simulink model "Sigma_Delta_NLDAC_DWA_RES_SL"  (Simulink 7.5)
settings: Solver=ode45  StartTime=0.0  StopTime=10.0  RelTol=1e-3
values from neighbouring files (symbols this model uses):
  a1 = 0.5019    [Loop_NLDAC.mat]    (also in Loop_NLDAC_BiDWA.mat; Sigma_Delta_Linear_DAC.m; Sigma_Delta_Linear_DAC_loop.m; Sigma_Delta_NLDAC.m)
  a2 = 0.3042    [Loop_NLDAC.mat]    (also in Loop_NLDAC_BiDWA.mat; Sigma_Delta_Linear_DAC.m; Sigma_Delta_Linear_DAC_loop.m; Sigma_Delta_NLDAC.m)
  alfa = 0.999    [Loop_NLDAC.mat]    (also in Loop_NLDAC_BiDWA.mat; Sigma_Delta_Linear_DAC.m; Sigma_Delta_Linear_DAC_loop.m; Sigma_Delta_NLDAC.m)
  Amax = 1.8    [Loop_NLDAC.mat]    (also in Loop_NLDAC_BiDWA.mat; Sigma_Delta_Linear_DAC.m; Sigma_Delta_Linear_DAC_loop.m; Sigma_Delta_NLDAC.m)
  Ampl = 0.19    [Loop_NLDAC.mat]    (also in Loop_NLDAC_BiDWA.mat; Sigma_Delta_Linear_DAC.m = 0.3; Sigma_Delta_Linear_DAC_loop.m; Sigma_Delta_NLDAC.m)
  b1 = 0.5019    [Loop_NLDAC.mat]    (also in Loop_NLDAC_BiDWA.mat; Sigma_Delta_Linear_DAC.m; Sigma_Delta_Linear_DAC_loop.m; Sigma_Delta_NLDAC.m)
  b2 = 0.3042    [Loop_NLDAC.mat]    (also in Loop_NLDAC_BiDWA.mat; Sigma_Delta_Linear_DAC.m; Sigma_Delta_Linear_DAC_loop.m; Sigma_Delta_NLDAC.m)
  b3 = 1    [Loop_NLDAC.mat]    (also in Loop_NLDAC_BiDWA.mat; Sigma_Delta_Linear_DAC.m = 0; Sigma_Delta_Linear_DAC_loop.m; Sigma_Delta_NLDAC.m)
  c1 = 0.2817    [Loop_NLDAC.mat]    (also in Loop_NLDAC_BiDWA.mat; Sigma_Delta_Linear_DAC.m; Sigma_Delta_Linear_DAC_loop.m; Sigma_Delta_NLDAC.m)
  c2 = 5.7104    [Loop_NLDAC.mat]    (also in Loop_NLDAC_BiDWA.mat; Sigma_Delta_Linear_DAC.m; Sigma_Delta_Linear_DAC_loop.m; Sigma_Delta_NLDAC.m)
  Cf = 2.5e-12    [Loop_NLDAC.mat]    (also in Loop_NLDAC_BiDWA.mat; Sigma_Delta_Linear_DAC.m; Sigma_Delta_Linear_DAC_loop.m; Sigma_Delta_NLDAC.m = 2.5)
  const = 0    [Loop_NLDAC.mat]    (also in Loop_NLDAC_BiDWA.mat; Sigma_Delta_Linear_DAC.m; Sigma_Delta_Linear_DAC_loop.m; Sigma_Delta_NLDAC.m)
  DAC_shift = 0.225    [Loop_NLDAC.mat]    (also in Loop_NLDAC_BiDWA.mat; Sigma_Delta_Linear_DAC.m; Sigma_Delta_Linear_DAC_loop.m; Sigma_Delta_NLDAC.m)
  finrad = 63.813600776    [Loop_NLDAC.mat]    (also in Loop_NLDAC_BiDWA.mat; Sigma_Delta_Linear_DAC.m = Fin*2*pi; Sigma_Delta_Linear_DAC_loop.m = Fin*2*pi; Sigma_Delta_NLDAC.m = Fin*2*pi)
  GBW = 4000000    [Loop_NLDAC.mat]    (also in Loop_NLDAC_BiDWA.mat; Sigma_Delta_Linear_DAC.m; Sigma_Delta_Linear_DAC_loop.m; Sigma_Delta_NLDAC.m)
  k = 1.38e-23    [Loop_NLDAC.mat]    (also in Loop_NLDAC_BiDWA.mat; Sigma_Delta_Linear_DAC.m; Sigma_Delta_Linear_DAC_loop.m; Sigma_Delta_NLDAC.m)
  noise1 = 3e-08    [Loop_NLDAC.mat]    (also in Loop_NLDAC_BiDWA.mat; Sigma_Delta_Linear_DAC.m; Sigma_Delta_Linear_DAC_loop.m; Sigma_Delta_NLDAC.m = 0)
  r1 = 0.5019    [Loop_NLDAC.mat]    (also in Loop_NLDAC_BiDWA.mat; Sigma_Delta_Linear_DAC.m; Sigma_Delta_Linear_DAC_loop.m; Sigma_Delta_NLDAC.m)
  r2 = 0.3042    [Loop_NLDAC.mat]    (also in Loop_NLDAC_BiDWA.mat; Sigma_Delta_Linear_DAC.m; Sigma_Delta_Linear_DAC_loop.m; Sigma_Delta_NLDAC.m)
  random = 0.1125    [Loop_NLDAC.mat]    (also in Loop_NLDAC_BiDWA.mat; Sigma_Delta_Linear_DAC.m; Sigma_Delta_Linear_DAC_loop.m; Sigma_Delta_NLDAC.m)
  sr = inf    [Loop_NLDAC.mat]    (also in Loop_NLDAC_BiDWA.mat; Sigma_Delta_Linear_DAC.m; Sigma_Delta_Linear_DAC_loop.m; Sigma_Delta_NLDAC.m)
  Temp = 300    [Loop_NLDAC.mat]    (also in Loop_NLDAC_BiDWA.mat; Sigma_Delta_Linear_DAC.m; Sigma_Delta_Linear_DAC_loop.m; Sigma_Delta_NLDAC.m)
  Ts = 1.953125e-05    [Loop_NLDAC.mat]    (also in Loop_NLDAC_BiDWA.mat; Sigma_Delta_Linear_DAC.m; Sigma_Delta_Linear_DAC_loop.m; Sigma_Delta_NLDAC.m)
  Ts_pn = Ts * 128    (= 0.0025)    [Sigma_Delta_NLDAC_DWA_RES.m]
  UEG0 = 0.225297400264    [Loop_NLDAC.mat]    (also in Loop_NLDAC_BiDWA.mat = 0.224094362454; Sigma_Delta_Linear_DAC_loop.m = DAC_step * ( 1 + frac_error(i,j,1) ); Sigma_Delta_NLDAC.m = DAC_step * ( 1 + frac_error(1) ); Sigma_Delta_NLDAC_BiDWA.m = DAC_step * ( 1 + frac_error(1) ))
  UEG1 = 0.225809869923    [Loop_NLDAC.mat]    (also in Loop_NLDAC_BiDWA.mat = 0.2240538032; Sigma_Delta_Linear_DAC_loop.m = DAC_step * ( 1 + frac_error(i,j,2) ); Sigma_Delta_NLDAC.m = DAC_step * ( 1 + frac_error(2) ); Sigma_Delta_NLDAC_BiDWA.m = DAC_step * ( 1 + frac_error(2) ))
  UEG2 = 0.224626431014    [Loop_NLDAC.mat]    (also in Loop_NLDAC_BiDWA.mat = 0.225728482718; Sigma_Delta_Linear_DAC_loop.m = DAC_step * ( 1 + frac_error(i,j,3) ); Sigma_Delta_NLDAC.m = DAC_step * ( 1 + frac_error(3) ); Sigma_Delta_NLDAC_BiDWA.m = DAC_step * ( 1 + frac_error(3) ))
  UEG3 = 0.225382310978    [Loop_NLDAC.mat]    (also in Loop_NLDAC_BiDWA.mat = 0.225896977376; Sigma_Delta_Linear_DAC_loop.m = DAC_step * ( 1 + frac_error(i,j,4) ); Sigma_Delta_NLDAC.m = DAC_step * ( 1 + frac_error(4) ); Sigma_Delta_NLDAC_BiDWA.m = DAC_step * ( 1 + frac_error(4) ))
  UEG4 = 0.225571027107    [Loop_NLDAC.mat]    (also in Loop_NLDAC_BiDWA.mat = 0.224420295179; Sigma_Delta_Linear_DAC_loop.m = DAC_step * ( 1 + frac_error(i,j,5) ); Sigma_Delta_NLDAC.m = DAC_step * ( 1 + frac_error(5) ); Sigma_Delta_NLDAC_BiDWA.m = DAC_step * ( 1 + frac_error(5) ))
  UEG5 = 0.225259624957    [Loop_NLDAC.mat]    (also in Loop_NLDAC_BiDWA.mat = 0.224828213498; Sigma_Delta_Linear_DAC_loop.m = DAC_step * ( 1 + frac_error(i,j,6) ); Sigma_Delta_NLDAC.m = DAC_step * ( 1 + frac_error(6) ); Sigma_Delta_NLDAC_BiDWA.m = DAC_step * ( 1 + frac_error(6) ))
  UEG6 = 0.224443920639    [Loop_NLDAC.mat]    (also in Loop_NLDAC_BiDWA.mat = 0.223228145386; Sigma_Delta_Linear_DAC_loop.m = DAC_step * ( 1 + frac_error(i,j,7) ); Sigma_Delta_NLDAC.m = DAC_step * ( 1 + frac_error(7) ); Sigma_Delta_NLDAC_BiDWA.m = DAC_step * ( 1 + frac_error(7) ))
  Vin_bias = 0.9    [Loop_NLDAC.mat]    (also in Loop_NLDAC_BiDWA.mat; Sigma_Delta_Linear_DAC.m; Sigma_Delta_Linear_DAC_loop.m; Sigma_Delta_NLDAC.m)
undefined symbols (not defined in the file or in its folder): clock, slew
libraries: simulink x8, commseqgen2 x2, simulink_extras x1
settings Model: Creator=test  LastModifiedBy=Mahmoud Sawaby

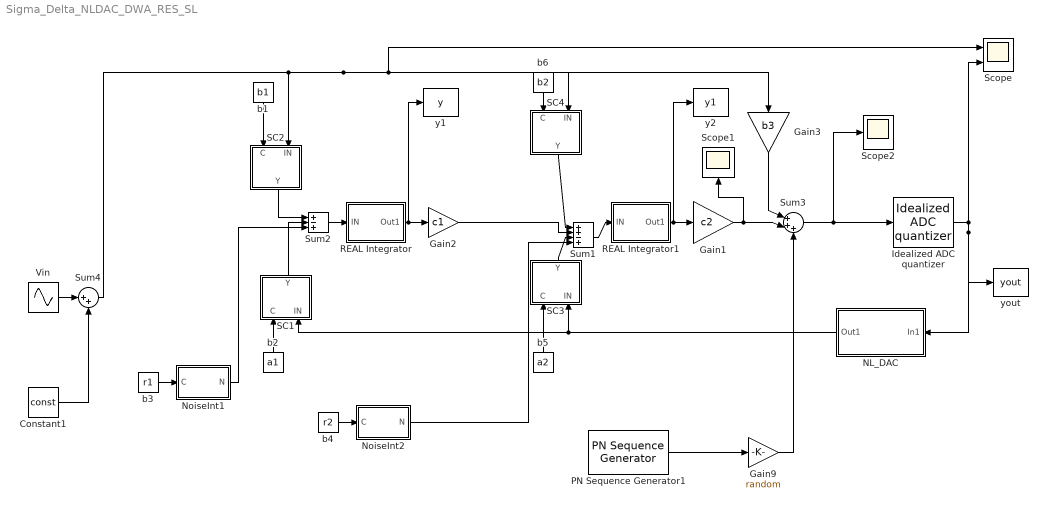
== system Sigma_Delta_NLDAC_DWA_RES_SL ==
  Constant1 : Constant  Value=const  OutDataType=fixdt(1, 16)  OutScaling=2^0  SampleTime=Ts
  Gain1 : Gain  Gain=c2  ParameterDataType=fixdt(1, 16)  ParameterScaling=2^0  OutDataType=fixdt(1, 16)  OutScaling=2^0
  Gain2 : Gain  Gain=c1  ParameterDataType=fixdt(1, 16)  ParameterScaling=2^0  OutDataType=fixdt(1, 16)  OutScaling=2^0
  Gain3 : Gain  Gain=b3  ParameterDataType=fixdt(1, 16)  ParameterScaling=2^0  OutDataType=fixdt(1, 16)  OutScaling=2^0
  Gain9 : Gain  Gain=random  ParameterDataType=fixdt(1, 16)  ParameterScaling=2^0  OutDataType=fixdt(1, 16)  OutScaling=2^0
  Idealized ADC quantizer : simulink_extras/Additional Discrete/Idealized ADC quantizer  SystemSampleTime=-1  NumberOfConverterBits=3  Vmin=MIN_volt  Vmax=MAX_volt  OutputDataType=double  OutputNegativeValues=off
  NL_DAC : Subsystem
  NoiseInt1 : Subsystem  mask(OpAmp Noise){seed=sum(clock)^1/111, Ts=Ts, noise=noise1}
      mask prompts: seed "Random Number Seed:"; Ts "Sample Time:"; noise "Op-amp Noise Std. Dev.:"
      mask Display: disp('OpNoise')
  NoiseInt2 : Subsystem  mask(OpAmp Noise){seed=sum(clock)^1/111, Ts=Ts, noise=noise1}
      mask prompts: seed "Random Number Seed:"; Ts "Sample Time:"; noise "Op-amp Noise Std. Dev.:"
      mask Display: disp('OpNoise')
  PN Sequence Generator1 : commseqgen2/PN Sequence Generator  poly=[1 0 0 0 0 0 0 0 0 0 0 1 0 1 1 0 1]  ini_sta=[0 0 0 0 0 0 0 0 0 0 0 0 0 0 0 1]  outBitMaskSource=Dialog parameter  shift=0  Ts=Ts  frameBased=off  sampPerFrame=18  reset=off  bitPackedOutputs=off  outDataType=double  numPackedBits=8  bitPackDataSigned=off  bitPackedOutDType=double
  REAL Integrator : Subsystem  mask(Integrator){Ts=Ts, alfa=alfa, Amax=Amax, sr=sr, GBW=GBW}
      mask prompts: Ts "Sample Time:"; alfa "Finite Gain:"; Amax "Saturation:"; sr "Slew Rate:"; GBW "Gain-Bandwidth"
      mask help:
      | Real discrete integrator with delay.
      | Models op-amp saturation and slew rate.
      mask Help:
      | Parameters:
      | Ts:       Sample time
      | G:         Finite op-amp gain (ideal op-amp G=1)
      | Amax:  Saturation value
      | sr:       slew rate in V/s
      mask Display: dpoly([0 1], [1 -1], 'z-')
  REAL Integrator1 : Subsystem  mask(Integrator){Ts=Ts, alfa=alfa, Amax=Amax, sr=sr, GBW=GBW}
      mask prompts: Ts "Sample Time:"; alfa "Finite Gain:"; Amax "Saturation:"; sr "Slew Rate:"; GBW "Gain-Bandwidth"
      mask help:
      | Real discrete integrator with delay.
      | Models op-amp saturation and slew rate.
      mask Help:
      | Parameters:
      | Ts:       Sample time
      | G:         Finite op-amp gain (ideal op-amp G=1)
      | Amax:  Saturation value
      | sr:       slew rate in V/s
      mask Display: dpoly([0 1], [1 -1], 'z-')
  SC1 : Subsystem  mask(kT/C Noise){Ts=Ts, Ci=Cf, Temp=Temp, k=k, seed=sum(clock)}
      mask prompts: Ts "Sample Time:"; Ci "Integrating Capacitance:"; Temp "Absolute Temperature:"; k "Boltzman Constant:"; seed "Random Number Seed:"
      mask help:
      | Models the kT/Cs noise of a switched capacitance Cs.
      | IN input: the input signal line
      | C input:   accepts the coefficient WITH SIGN (Cs/Ci)
      mask Help:
      | Block parameters:
      | Ts:        Sample time
      | Ci:        Integrating Capacitance
      | Temp:   Absolute Temperature in Kelvin
      | k:         Boltzmann Constant
      | seed:    Initial seed for random number generator
      | Outputs the noisy signal.
      mask Display: disp('kT/C')
  SC2 : Subsystem  mask(kT/C Noise){Ts=Ts, Ci=Cf, Temp=Temp, k=k, seed=sum(clock)}
      mask prompts: Ts "Sample Time:"; Ci "Integrating Capacitance:"; Temp "Absolute Temperature:"; k "Boltzman Constant:"; seed "Random Number Seed:"
      mask help:
      | Models the kT/Cs noise of a switched capacitance Cs.
      | IN input: the input signal line
      | C input:   accepts the coefficient WITH SIGN (Cs/Ci)
      mask Help:
      | Block parameters:
      | Ts:        Sample time
      | Ci:        Integrating Capacitance
      | Temp:   Absolute Temperature in Kelvin
      | k:         Boltzmann Constant
      | seed:    Initial seed for random number generator
      | Outputs the noisy signal.
      mask Display: disp('kT/C')
  SC3 : Subsystem  mask(kT/C Noise){Ts=Ts, Ci=Cf, Temp=Temp, k=k, seed=sum(clock)}
      mask prompts: Ts "Sample Time:"; Ci "Integrating Capacitance:"; Temp "Absolute Temperature:"; k "Boltzman Constant:"; seed "Random Number Seed:"
      mask help:
      | Models the kT/Cs noise of a switched capacitance Cs.
      | IN input: the input signal line
      | C input:   accepts the coefficient WITH SIGN (Cs/Ci)
      mask Help:
      | Block parameters:
      | Ts:        Sample time
      | Ci:        Integrating Capacitance
      | Temp:   Absolute Temperature in Kelvin
      | k:         Boltzmann Constant
      | seed:    Initial seed for random number generator
      | Outputs the noisy signal.
      mask Display: disp('kT/C')
  SC4 : Subsystem  mask(kT/C Noise){Ts=Ts, Ci=Cf, Temp=Temp, k=k, seed=sum(clock)}
      mask prompts: Ts "Sample Time:"; Ci "Integrating Capacitance:"; Temp "Absolute Temperature:"; k "Boltzman Constant:"; seed "Random Number Seed:"
      mask help:
      | Models the kT/Cs noise of a switched capacitance Cs.
      | IN input: the input signal line
      | C input:   accepts the coefficient WITH SIGN (Cs/Ci)
      mask Help:
      | Block parameters:
      | Ts:        Sample time
      | Ci:        Integrating Capacitance
      | Temp:   Absolute Temperature in Kelvin
      | k:         Boltzmann Constant
      | seed:    Initial seed for random number generator
      | Outputs the noisy signal.
      mask Display: disp('kT/C')
  Scope : Scope  NumInputPorts=2
      settings: YMin=0.1~-1  YMax=1.7~8  MaxDataPoints=65536
  Scope1 : Scope
  Scope2 : Scope
      settings: YMin=-0.5  YMax=2.4  SaveName=ScopeData2  MaxDataPoints=65536
  Sum1 : Sum  Inputs=++-+  SaturateOnIntegerOverflow=on  InputSameDT=on  OutDataTypeStr=Inherit: Same as first input
  Sum2 : Sum  Inputs=+-+  SaturateOnIntegerOverflow=on  InputSameDT=on  OutDataTypeStr=Inherit: Same as first input
  Sum3 : Sum  Inputs=|+++  OutDataType=fixdt(1, 16)  OutScaling=2^0
  Sum4 : Sum  Inputs=|++  OutDataType=fixdt(1, 16)  OutScaling=2^0
  Vin : Sin  Amplitude=Ampl  Bias=Vin_bias  Frequency=finrad  Phase=0  Samples=10  SampleTime=Ts  Offset=0
  b1 : Constant  Value=b1  SampleTime=Ts
  b2 : Constant  Value=a1  SampleTime=Ts
  b3 : Constant  Value=r1
  b4 : Constant  Value=r2
  b5 : Constant  Value=a2  SampleTime=Ts
  b6 : Constant  Value=b2  SampleTime=Ts
  y1 : ToWorkspace  VariableName=y  SampleTime=-1  SaveFormat=Array
  y2 : ToWorkspace  VariableName=y1  SampleTime=-1  SaveFormat=Array
  yout : ToWorkspace  VariableName=yout  SampleTime=Ts  SaveFormat=Array
  wires:
  Idealized ADC quantizer/1 -> yout/1, NL_DAC/1(In1), Scope/2
  Gain1/1 -> Scope1/1, Sum3/2
  REAL Integrator/1(Out1) -> y1/1, Gain2/1
  REAL Integrator1/1(Out1) -> Gain1/1, y2/1
  Sum2/1 -> REAL Integrator/1(IN)
  Sum3/1 -> Idealized ADC quantizer/1, Scope2/1
  Gain3/1 -> Sum3/1
  Sum4/1 -> Scope/1, Gain3/1, SC4/2(IN), SC2/2(IN)
  Constant1/1 -> Sum4/2
  Gain9/1 -> Sum3/3
  Vin/1 -> Sum4/1
  SC1/1(Y) -> Sum2/2
  b2/1 -> SC1/1(C)
  b1/1 -> SC2/1(C)
  SC2/1(Y) -> Sum2/1
  SC4/1(Y) -> Sum1/1
  Gain2/1 -> Sum1/2
  SC3/1(Y) -> Sum1/3
  Sum1/1 -> REAL Integrator1/1(IN)
  PN Sequence Generator1/1 -> Gain9/1
  b3/1 -> NoiseInt1/1(C)
  NoiseInt1/1(N) -> Sum2/3
  b4/1 -> NoiseInt2/1(C)
  b5/1 -> SC3/1(C)
  b6/1 -> SC4/1(C)
  NL_DAC/1(Out1) -> SC1/2(IN), SC3/2(IN)
  NoiseInt2/1(N) -> Sum1/4

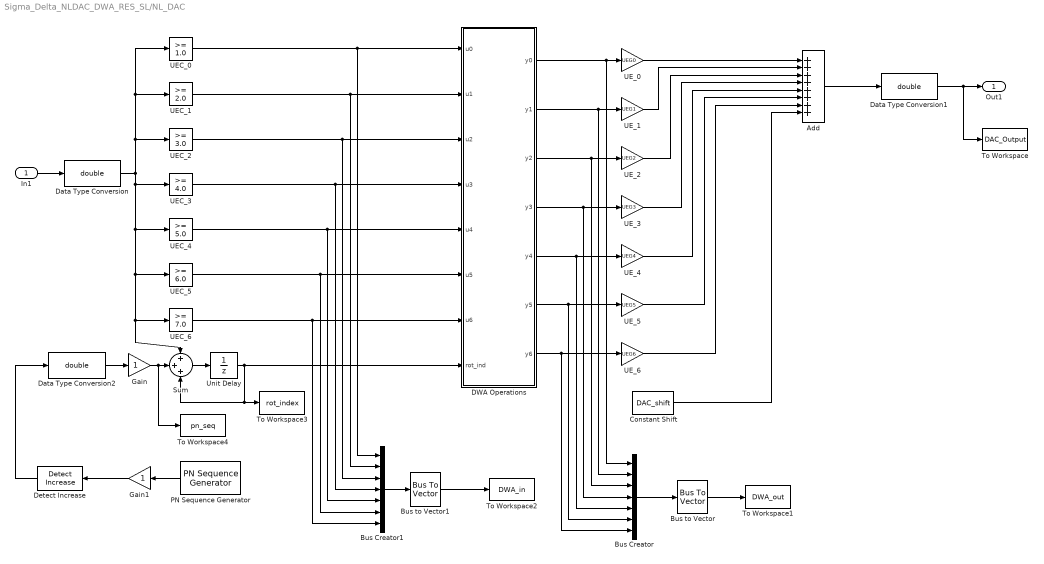
== system Sigma_Delta_NLDAC_DWA_RES_SL/NL_DAC ==
  In1 : Inport  OutDataType=fixdt(1, 16)  OutScaling=2^0
  Add : Sum  Inputs=++++++++  OutDataType=fixdt(1, 16)  OutScaling=2^-10
  Bus Creator : BusCreator  Inputs=7
  Bus Creator1 : BusCreator  Inputs=7
  Bus to Vector : BusToVector
  Bus to Vector1 : BusToVector
  Constant Shift : Constant  Value=DAC_shift  OutDataType=fixdt(1, 16)  OutScaling=2^0  SampleTime=Ts
  DWA Operations : Stateflow chart  TreatAsAtomicUnit=on  SystemSampleTime=Ts
  Data Type Conversion : DataTypeConversion  OutDataTypeMode=double  OutDataType=fixdt(1, 16)  OutScaling=2^0  OutDataTypeStr=double  SampleTime=Ts
  Data Type Conversion1 : DataTypeConversion  OutDataTypeMode=double  OutDataType=fixdt(1, 16)  OutScaling=2^0  OutDataTypeStr=double
  Data Type Conversion2 : DataTypeConversion  OutDataTypeMode=double  OutDataType=fixdt(1, 16)  OutScaling=2^0  OutDataTypeStr=double  SampleTime=Ts
  Detect Increase : simulink/Logic and Bit Operations/Detect Increase  SystemSampleTime=-1  vinit=0.0
  Gain : Gain  ParameterDataType=fixdt(1, 16)  ParameterScaling=2^0  OutDataType=fixdt(1, 16)  OutScaling=2^0
  Gain1 : Gain  ParameterDataType=fixdt(1, 16)  ParameterScaling=2^0  OutDataType=fixdt(1, 16)  OutScaling=2^0  SampleTime=Ts
  PN Sequence Generator : commseqgen2/PN Sequence Generator  poly=[6 5 0]  ini_sta=[0 0 0 0 0 1]  outBitMaskSource=Dialog parameter  shift=0  Ts=Ts_pn  frameBased=off  sampPerFrame=1  reset=off  bitPackedOutputs=off  outDataType=double  numPackedBits=8  bitPackDataSigned=off  bitPackedOutDType=double
  Sum : Sum  Inputs=+++  OutDataType=fixdt(1, 16)  OutScaling=2^0
  To Workspace : ToWorkspace  VariableName=DAC_Output  SampleTime=-1  SaveFormat=Array
  To Workspace1 : ToWorkspace  VariableName=DWA_out  SampleTime=-1  SaveFormat=Array
  To Workspace2 : ToWorkspace  VariableName=DWA_in  SampleTime=-1  SaveFormat=Array
  To Workspace3 : ToWorkspace  VariableName=rot_index  SampleTime=-1  SaveFormat=Array
  To Workspace4 : ToWorkspace  VariableName=pn_seq  SampleTime=-1  SaveFormat=Array
  UEC_0 : simulink/Logic and Bit Operations/Compare To Constant  SystemSampleTime=-1  relop=>=  const=1.0  LogicOutDataTypeMode=uint8
  UEC_1 : simulink/Logic and Bit Operations/Compare To Constant  SystemSampleTime=-1  relop=>=  const=2.0  LogicOutDataTypeMode=uint8
  UEC_2 : simulink/Logic and Bit Operations/Compare To Constant  SystemSampleTime=-1  relop=>=  const=3.0  LogicOutDataTypeMode=uint8
  UEC_3 : simulink/Logic and Bit Operations/Compare To Constant  SystemSampleTime=-1  relop=>=  const=4.0  LogicOutDataTypeMode=uint8
  UEC_4 : simulink/Logic and Bit Operations/Compare To Constant  SystemSampleTime=-1  relop=>=  const=5.0  LogicOutDataTypeMode=uint8
  UEC_5 : simulink/Logic and Bit Operations/Compare To Constant  SystemSampleTime=-1  relop=>=  const=6.0  LogicOutDataTypeMode=uint8
  UEC_6 : simulink/Logic and Bit Operations/Compare To Constant  SystemSampleTime=-1  relop=>=  const=7.0  LogicOutDataTypeMode=uint8
  UE_0 : Gain  Gain=UEG0  ParameterDataType=fixdt(1, 16)  ParameterScaling=2^0  OutDataType=fixdt(1, 16)  OutScaling=2^0
  UE_1 : Gain  Gain=UEG1  ParameterDataType=fixdt(1, 16)  ParameterScaling=2^0  OutDataType=fixdt(1, 16)  OutScaling=2^0
  UE_2 : Gain  Gain=UEG2  ParameterDataType=fixdt(1, 16)  ParameterScaling=2^0  OutDataType=fixdt(1, 16)  OutScaling=2^0
  UE_3 : Gain  Gain=UEG3  ParameterDataType=fixdt(1, 16)  ParameterScaling=2^0  OutDataType=fixdt(1, 16)  OutScaling=2^0
  UE_4 : Gain  Gain=UEG4  ParameterDataType=fixdt(1, 16)  ParameterScaling=2^0  OutDataType=fixdt(1, 16)  OutScaling=2^0
  UE_5 : Gain  Gain=UEG5  ParameterDataType=fixdt(1, 16)  ParameterScaling=2^0  OutDataType=fixdt(1, 16)  OutScaling=2^0
  UE_6 : Gain  Gain=UEG6  ParameterDataType=fixdt(1, 16)  ParameterScaling=2^0  OutDataType=fixdt(1, 16)  OutScaling=2^0
  Unit Delay : UnitDelay  SampleTime=-1
  Out1 : Outport  OutDataType=fixdt(1, 16)  OutScaling=2^0
  wires:
  UE_0/1 -> Add/1
  UE_1/1 -> Add/2
  UE_2/1 -> Add/3
  UE_3/1 -> Add/4
  UE_4/1 -> Add/5
  UE_5/1 -> Add/6
  UE_6/1 -> Add/7
  Data Type Conversion/1 -> UEC_0/1, UEC_1/1, UEC_2/1, UEC_5/1, UEC_6/1, Sum/1, UEC_4/1, UEC_3/1
  In1/1 -> Data Type Conversion/1
  Add/1 -> Data Type Conversion1/1
  Data Type Conversion1/1 -> Out1/1, To Workspace/1
  Constant Shift/1 -> Add/8
  UEC_0/1 -> DWA Operations/1(u0), Bus Creator1/1
  UEC_1/1 -> DWA Operations/2(u1), Bus Creator1/2
  UEC_2/1 -> DWA Operations/3(u2), Bus Creator1/3
  UEC_3/1 -> DWA Operations/4(u3), Bus Creator1/4
  UEC_4/1 -> DWA Operations/5(u4), Bus Creator1/5
  UEC_5/1 -> DWA Operations/6(u5), Bus Creator1/6
  UEC_6/1 -> DWA Operations/7(u6), Bus Creator1/7
  DWA Operations/1(y0) -> UE_0/1, Bus Creator/1
  DWA Operations/2(y1) -> UE_1/1, Bus Creator/2
  DWA Operations/3(y2) -> UE_2/1, Bus Creator/3
  DWA Operations/4(y3) -> UE_3/1, Bus Creator/4
  DWA Operations/5(y4) -> UE_4/1, Bus Creator/5
  DWA Operations/6(y5) -> UE_5/1, Bus Creator/6
  DWA Operations/7(y6) -> UE_6/1, Bus Creator/7
  Bus Creator/1 -> Bus to Vector/1
  Bus to Vector/1 -> To Workspace1/1
  Bus Creator1/1 -> Bus to Vector1/1
  Bus to Vector1/1 -> To Workspace2/1
  Sum/1 -> Unit Delay/1
  Unit Delay/1 -> DWA Operations/8(rot_ind), To Workspace3/1, Sum/3
  Detect Increase/1 -> Data Type Conversion2/1
  Data Type Conversion2/1 -> Gain/1
  Gain/1 -> Sum/2, To Workspace4/1
  PN Sequence Generator/1 -> Gain1/1
  Gain1/1 -> Detect Increase/1

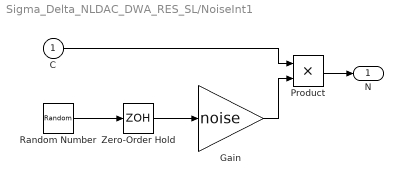
== system Sigma_Delta_NLDAC_DWA_RES_SL/NoiseInt1 ==
  C : Inport
  Gain : Gain  Gain=noise  SaturateOnIntegerOverflow=on  OutDataTypeStr=Inherit: Same as input  ParamDataTypeStr=Inherit: Same as input
  Product : Product  SaturateOnIntegerOverflow=on  RndMeth=Zero  InputSameDT=on  OutDataTypeStr=Inherit: Same as first input
  Random Number : RandomNumber  Seed=seed  SampleTime=Ts
  Zero-Order Hold : ZeroOrderHold  SampleTime=Ts
  N : Outport  InitialOutput=0
  wires:
  Random Number/1 -> Zero-Order Hold/1
  Zero-Order Hold/1 -> Gain/1
  Product/1 -> N/1
  Gain/1 -> Product/2
  C/1 -> Product/1

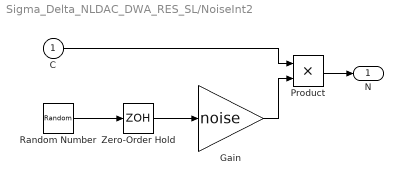
== system Sigma_Delta_NLDAC_DWA_RES_SL/NoiseInt2 ==
  C : Inport
  Gain : Gain  Gain=noise  SaturateOnIntegerOverflow=on  OutDataTypeStr=Inherit: Same as input  ParamDataTypeStr=Inherit: Same as input
  Product : Product  SaturateOnIntegerOverflow=on  RndMeth=Zero  InputSameDT=on  OutDataTypeStr=Inherit: Same as first input
  Random Number : RandomNumber  Seed=seed  SampleTime=Ts
  Zero-Order Hold : ZeroOrderHold  SampleTime=Ts
  N : Outport  InitialOutput=0
  wires:
  Random Number/1 -> Zero-Order Hold/1
  Zero-Order Hold/1 -> Gain/1
  Product/1 -> N/1
  Gain/1 -> Product/2
  C/1 -> Product/1

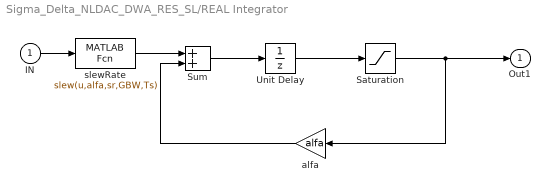
== system Sigma_Delta_NLDAC_DWA_RES_SL/REAL Integrator ==
  IN : Inport
  Saturation : Saturate  UpperLimit=Amax  LowerLimit=-Amax
  Sum : Sum  SaturateOnIntegerOverflow=on  InputSameDT=on  OutDataTypeStr=Inherit: Same as first input
  Unit Delay : UnitDelay  SampleTime=Ts
  alfa : Gain  Gain=alfa  SaturateOnIntegerOverflow=on  OutDataTypeStr=Inherit: Same as input  ParamDataTypeStr=Inherit: Same as input
  slewRate : MATLABFcn  MATLABFcn=slew(u,alfa,sr,GBW,Ts)
  Out1 : Outport
  wires:
  Sum/1 -> Unit Delay/1
  Unit Delay/1 -> Saturation/1
  Saturation/1 -> Out1/1, alfa/1
  IN/1 -> slewRate/1
  slewRate/1 -> Sum/1
  alfa/1 -> Sum/2

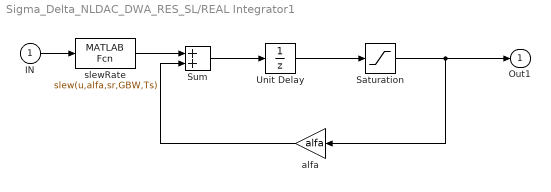
== system Sigma_Delta_NLDAC_DWA_RES_SL/REAL Integrator1 ==
  IN : Inport
  Saturation : Saturate  UpperLimit=Amax  LowerLimit=-Amax
  Sum : Sum  SaturateOnIntegerOverflow=on  InputSameDT=on  OutDataTypeStr=Inherit: Same as first input
  Unit Delay : UnitDelay  SampleTime=Ts
  alfa : Gain  Gain=alfa  SaturateOnIntegerOverflow=on  OutDataTypeStr=Inherit: Same as input  ParamDataTypeStr=Inherit: Same as input
  slewRate : MATLABFcn  MATLABFcn=slew(u,alfa,sr,GBW,Ts)
  Out1 : Outport
  wires:
  Sum/1 -> Unit Delay/1
  Unit Delay/1 -> Saturation/1
  Saturation/1 -> Out1/1, alfa/1
  IN/1 -> slewRate/1
  slewRate/1 -> Sum/1
  alfa/1 -> Sum/2

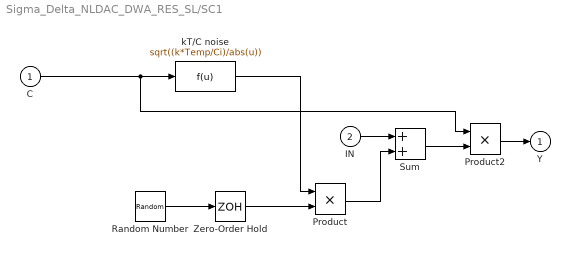
== system Sigma_Delta_NLDAC_DWA_RES_SL/SC1 ==
  C : Inport
  IN : Inport  Port=2
  Product : Product  SaturateOnIntegerOverflow=on  RndMeth=Zero  InputSameDT=on  OutDataTypeStr=Inherit: Same as first input
  Product2 : Product  SaturateOnIntegerOverflow=on  RndMeth=Zero  InputSameDT=on  OutDataTypeStr=Inherit: Same as first input
  Random Number : RandomNumber  Seed=seed  SampleTime=Ts
  Sum : Sum  SaturateOnIntegerOverflow=on  InputSameDT=on  OutDataTypeStr=Inherit: Same as first input
  Zero-Order Hold : ZeroOrderHold  SampleTime=Ts
  kT/C noise : Fcn  Expr=sqrt((k*Temp/Ci)/abs(u))
  Y : Outport  InitialOutput=0
  wires:
  Random Number/1 -> Zero-Order Hold/1
  C/1 -> Product2/1, kT/C noise/1
  Zero-Order Hold/1 -> Product/2
  kT/C noise/1 -> Product/1
  Sum/1 -> Product2/2
  IN/1 -> Sum/1
  Product2/1 -> Y/1
  Product/1 -> Sum/2

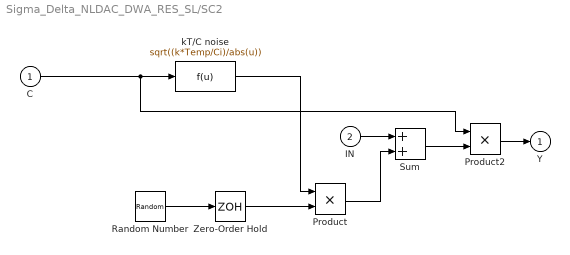
== system Sigma_Delta_NLDAC_DWA_RES_SL/SC2 ==
  C : Inport
  IN : Inport  Port=2
  Product : Product  SaturateOnIntegerOverflow=on  RndMeth=Zero  InputSameDT=on  OutDataTypeStr=Inherit: Same as first input
  Product2 : Product  SaturateOnIntegerOverflow=on  RndMeth=Zero  InputSameDT=on  OutDataTypeStr=Inherit: Same as first input
  Random Number : RandomNumber  Seed=seed  SampleTime=Ts
  Sum : Sum  SaturateOnIntegerOverflow=on  InputSameDT=on  OutDataTypeStr=Inherit: Same as first input
  Zero-Order Hold : ZeroOrderHold  SampleTime=Ts
  kT/C noise : Fcn  Expr=sqrt((k*Temp/Ci)/abs(u))
  Y : Outport  InitialOutput=0
  wires:
  Random Number/1 -> Zero-Order Hold/1
  C/1 -> Product2/1, kT/C noise/1
  Zero-Order Hold/1 -> Product/2
  kT/C noise/1 -> Product/1
  Sum/1 -> Product2/2
  IN/1 -> Sum/1
  Product2/1 -> Y/1
  Product/1 -> Sum/2

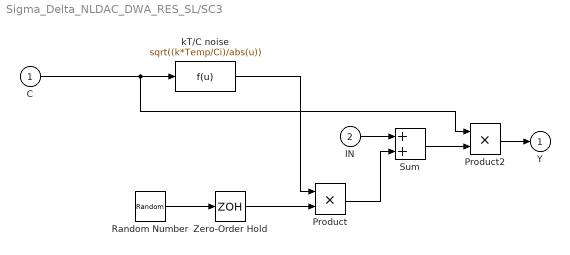
== system Sigma_Delta_NLDAC_DWA_RES_SL/SC3 ==
  C : Inport
  IN : Inport  Port=2
  Product : Product  SaturateOnIntegerOverflow=on  RndMeth=Zero  InputSameDT=on  OutDataTypeStr=Inherit: Same as first input
  Product2 : Product  SaturateOnIntegerOverflow=on  RndMeth=Zero  InputSameDT=on  OutDataTypeStr=Inherit: Same as first input
  Random Number : RandomNumber  Seed=seed  SampleTime=Ts
  Sum : Sum  SaturateOnIntegerOverflow=on  InputSameDT=on  OutDataTypeStr=Inherit: Same as first input
  Zero-Order Hold : ZeroOrderHold  SampleTime=Ts
  kT/C noise : Fcn  Expr=sqrt((k*Temp/Ci)/abs(u))
  Y : Outport  InitialOutput=0
  wires:
  Random Number/1 -> Zero-Order Hold/1
  C/1 -> Product2/1, kT/C noise/1
  Zero-Order Hold/1 -> Product/2
  kT/C noise/1 -> Product/1
  Sum/1 -> Product2/2
  IN/1 -> Sum/1
  Product2/1 -> Y/1
  Product/1 -> Sum/2

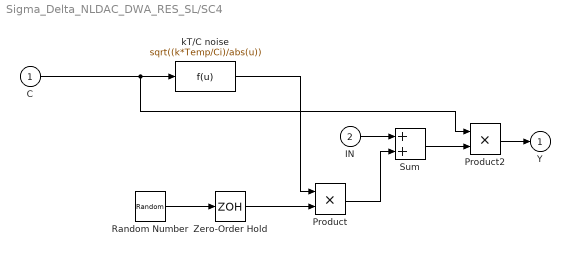
== system Sigma_Delta_NLDAC_DWA_RES_SL/SC4 ==
  C : Inport
  IN : Inport  Port=2
  Product : Product  SaturateOnIntegerOverflow=on  RndMeth=Zero  InputSameDT=on  OutDataTypeStr=Inherit: Same as first input
  Product2 : Product  SaturateOnIntegerOverflow=on  RndMeth=Zero  InputSameDT=on  OutDataTypeStr=Inherit: Same as first input
  Random Number : RandomNumber  Seed=seed  SampleTime=Ts
  Sum : Sum  SaturateOnIntegerOverflow=on  InputSameDT=on  OutDataTypeStr=Inherit: Same as first input
  Zero-Order Hold : ZeroOrderHold  SampleTime=Ts
  kT/C noise : Fcn  Expr=sqrt((k*Temp/Ci)/abs(u))
  Y : Outport  InitialOutput=0
  wires:
  Random Number/1 -> Zero-Order Hold/1
  C/1 -> Product2/1, kT/C noise/1
  Zero-Order Hold/1 -> Product/2
  kT/C noise/1 -> Product/1
  Sum/1 -> Product2/2
  IN/1 -> Sum/1
  Product2/1 -> Y/1
  Product/1 -> Sum/2

== matlab function NL_DAC/DWA Operations ==
  data: u0 input double; y0 output double; u1 input double; y1 output double; y2 output double; u2 input double; u3 input double; u4 input double; u5 input double; u6 input double; y3 output double; y4 output double; y5 output double; y6 output double; rot_ind input double
function [y0,y1,y2,y3,y4,y5,y6] = dwa(u0,u1,u2,u3,u4,u5,u6,rot_ind)
%#eml

eml.extrinsic('dwa_function');
y0 = 0;
y1 = 0;
y2 = 0;
y3 = 0;
y4 = 0;
y5 = 0;
y6 = 0;
[y0,y1,y2,y3,y4,y5,y6] = dwa_function(u0,u1,u2,u3,u4,u5,u6,rot_ind);
